simulink model "ref_sim"  (R2025b)
settings: Solver=VariableStepAuto  StartTime=0.0  StopTime=10.0  RelTol=1e-3
undefined symbols (not defined in the file or in its folder): none
libraries: imaqlib x1
settings Model: Creator=kazuh  LastModifiedBy=kazuh

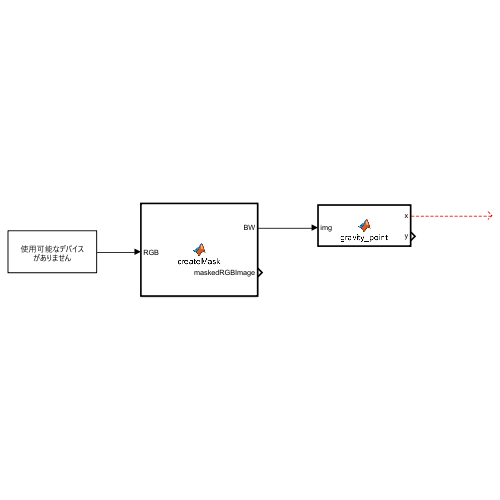
[thumbnail: Simulink's stored preview of the top-level diagram]
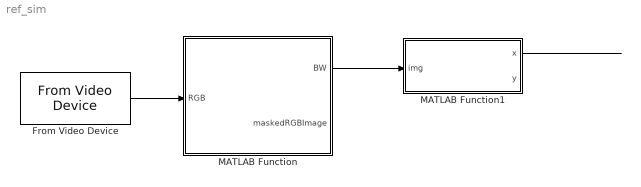
== system ref_sim ==
  From Video Device : imaqlib/From Video Device  DeviceMenu=(none)  Device=(none)  ObjConstructor=(none)  VideoFormatMenu=(none)  VideoFormat=(none)  VideoSource=none  ROIPosition=(none)  EnableHWTrigger=off  TriggerConfiguration=none/none  SampleTime=1/30  OutputPortsMode=One multidimensional signal  DataType=single  CanDoHWTrigger=no  ReturnedColorSpace=rgb  BlockHandle=157.0002  ROIWidth=100  ROIHeight=100  ROIColumn=0  ROIRow=0  EngXMLPath=C:\Program Files\MATLAB\R2025b\toolbox\imaq\imaq\private  DevXMLPath=DEVPATH  EngLibPath=C:\Program Files\MATLAB\R2025b\toolbox\imaq\imaqblks\imaqmex\win64  ColorSpace=rgb  BayerSensorAlignment=grbg  ImaqMode=off
  MATLAB Function : MATLAB Function  TreatAsAtomicUnit=on
  MATLAB Function1 : MATLAB Function  TreatAsAtomicUnit=on
  wires:
  From Video Device/1 -> MATLAB Function/1(RGB)
  MATLAB Function/1(BW) -> MATLAB Function1/1(img)
  MATLAB Function1/1(x) -> ?

== matlab function ref_sim/MATLAB Function ==
  data: RGB input; BW output; maskedRGBImage output
function [BW,maskedRGBImage] = createMask(RGB)
%createMask  Threshold RGB image using auto-generated code from colorThresholder app.
%  [BW,MASKEDRGBIMAGE] = createMask(RGB) thresholds image RGB using
%  auto-generated code from the colorThresholder app. The colorspace and
%  range for each channel of the colorspace were set within the app. The
%  segmentation mask is returned in BW, and a composite of the mask and
%  original RGB images is returned in maskedRGBImage.

% Auto-generated by colorThresholder app on 07-May-2026
%------------------------------------------------------


% Convert RGB image to chosen color space
I = rgb2hsv(RGB);

% Define thresholds for channel 1 based on histogram settings
channel1Min = 0;
channel1Max = 80/255;

% Define thresholds for channel 2 based on histogram settings
channel2Min = 90/255;
channel2Max = 1;

% Define thresholds for channel 3 based on histogram settings
channel3Min = 100/255;
channel3Max = 1;

% Create mask based on chosen histogram thresholds
sliderBW = (I(:,:,1) >= channel1Min ) & (I(:,:,1) <= channel1Max) & ...
    (I(:,:,2) >= channel2Min ) & (I(:,:,2) <= channel2Max) & ...
    (I(:,:,3) >= channel3Min ) & (I(:,:,3) <= channel3Max);
BW = sliderBW;

% Initialize output masked image based on input image.
maskedRGBImage = RGB;

% Set background pixels where BW is false to zero.
maskedRGBImage(repmat(~BW,[1 1 3])) = 0;

end

== matlab function ref_sim/MATLAB Function1 ==
  data: x output; img input; y output
function [x,y] = gravity_point(img)
[x_size, y_size] = size(img);
x_pos = 1:x_size;
y_pos = 1:y_size;

x_all = 0;
y_all = 0;

for i = y_pos
    x_all = x_all + sum((img(:,i) .* (x_pos)'))/sum(img(:,i));
end
x = mean(x_all)/x_size;

for i = x_pos
    y_all = y_all + sum((img(i,:) .* (y_pos)'))/sum(img(i,:));
end
y = mean(y_all)/y_size;
